simulink model "parallel_phase_voltages_per_switching_state_6"  (R2022a)
settings: Solver=FixedStepDiscrete  StartTime=0.0  StopTime=10.0  RelTol=1e-3
values from neighbouring files (symbols this model uses):
  f_c = 100000    [MPC_params.m]
  Rt = 1e-8    (= 1e-08)    [MPC_params.m]
  u_dc = 565    [MPC_params.m]
libraries: simulink x2, hdlsllib x2
(part 2 of 4)

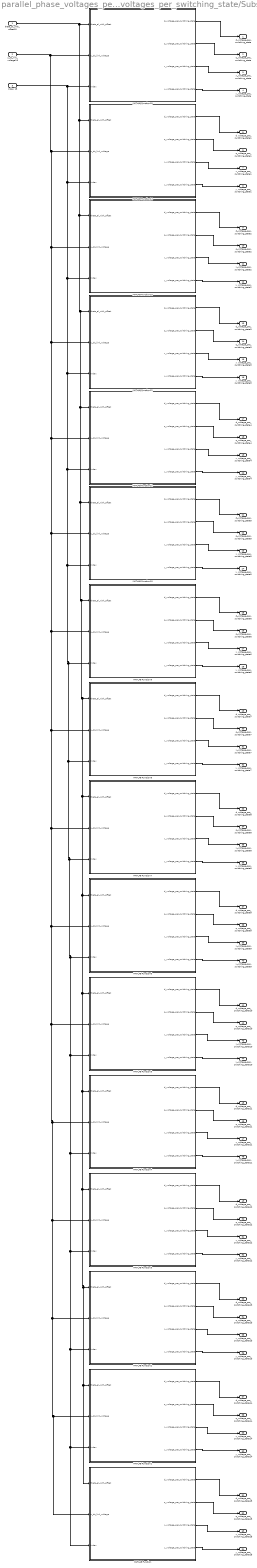
== system parallel_phase_voltages_per_switching_state_6/Phase_voltages_per_switching_state/Subsystem ==
  theta_el_with_offset15 : Inport
  u_dc_link_voltage15 : Inport  Port=2
  Index 15 : Inport  Port=3
  MATLAB Function : MATLAB Function  TreatAsAtomicUnit=on
  MATLAB Function1 : MATLAB Function  TreatAsAtomicUnit=on
  MATLAB Function10 : MATLAB Function  TreatAsAtomicUnit=on
  MATLAB Function11 : MATLAB Function  TreatAsAtomicUnit=on
  MATLAB Function12 : MATLAB Function  TreatAsAtomicUnit=on
  MATLAB Function13 : MATLAB Function  TreatAsAtomicUnit=on
  MATLAB Function14 : MATLAB Function  TreatAsAtomicUnit=on
  MATLAB Function15 : MATLAB Function  TreatAsAtomicUnit=on
  MATLAB Function2 : MATLAB Function  TreatAsAtomicUnit=on
  MATLAB Function3 : MATLAB Function  TreatAsAtomicUnit=on
  MATLAB Function4 : MATLAB Function  TreatAsAtomicUnit=on
  MATLAB Function5 : MATLAB Function  TreatAsAtomicUnit=on
  MATLAB Function6 : MATLAB Function  TreatAsAtomicUnit=on
  MATLAB Function7 : MATLAB Function  TreatAsAtomicUnit=on
  MATLAB Function8 : MATLAB Function  TreatAsAtomicUnit=on
  MATLAB Function9 : MATLAB Function  TreatAsAtomicUnit=on
  d_voltage_per_switching_state : Outport
  q_voltage_per_switching_state : Outport  Port=2
  x_voltage_per_switching_state : Outport  Port=3
  y_voltage_per_switching_state : Outport  Port=4
  d_voltage_per_switching_state1 : Outport  Port=5
  q_voltage_per_switching_state1 : Outport  Port=6
  x_voltage_per_switching_state1 : Outport  Port=7
  y_voltage_per_switching_state1 : Outport  Port=8
  d_voltage_per_switching_state2 : Outport  Port=9
  q_voltage_per_switching_state2 : Outport  Port=10
  x_voltage_per_switching_state2 : Outport  Port=11
  y_voltage_per_switching_state2 : Outport  Port=12
  d_voltage_per_switching_state3 : Outport  Port=13
  q_voltage_per_switching_state3 : Outport  Port=14
  x_voltage_per_switching_state3 : Outport  Port=15
  y_voltage_per_switching_state3 : Outport  Port=16
  d_voltage_per_switching_state4 : Outport  Port=17
  q_voltage_per_switching_state4 : Outport  Port=18
  x_voltage_per_switching_state4 : Outport  Port=19
  y_voltage_per_switching_state4 : Outport  Port=20
  d_voltage_per_switching_state5 : Outport  Port=21
  q_voltage_per_switching_state5 : Outport  Port=22
  x_voltage_per_switching_state5 : Outport  Port=23
  y_voltage_per_switching_state5 : Outport  Port=24
  d_voltage_per_switching_state6 : Outport  Port=25
  q_voltage_per_switching_state6 : Outport  Port=26
  x_voltage_per_switching_state6 : Outport  Port=27
  y_voltage_per_switching_state6 : Outport  Port=28
  d_voltage_per_switching_state7 : Outport  Port=29
  q_voltage_per_switching_state7 : Outport  Port=30
  x_voltage_per_switching_state7 : Outport  Port=31
  y_voltage_per_switching_state7 : Outport  Port=32
  d_voltage_per_switching_state8 : Outport  Port=33
  q_voltage_per_switching_state8 : Outport  Port=34
  x_voltage_per_switching_state8 : Outport  Port=35
  y_voltage_per_switching_state8 : Outport  Port=36
  d_voltage_per_switching_state9 : Outport  Port=37
  q_voltage_per_switching_state9 : Outport  Port=38
  x_voltage_per_switching_state9 : Outport  Port=39
  y_voltage_per_switching_state9 : Outport  Port=40
  d_voltage_per_switching_state10 : Outport  Port=41
  q_voltage_per_switching_state10 : Outport  Port=42
  x_voltage_per_switching_state10 : Outport  Port=43
  y_voltage_per_switching_state10 : Outport  Port=44
  d_voltage_per_switching_state11 : Outport  Port=45
  q_voltage_per_switching_state11 : Outport  Port=46
  x_voltage_per_switching_state11 : Outport  Port=47
  y_voltage_per_switching_state11 : Outport  Port=48
  d_voltage_per_switching_state12 : Outport  Port=49
  q_voltage_per_switching_state12 : Outport  Port=50
  x_voltage_per_switching_state12 : Outport  Port=51
  y_voltage_per_switching_state12 : Outport  Port=52
  d_voltage_per_switching_state13 : Outport  Port=53
  q_voltage_per_switching_state13 : Outport  Port=54
  x_voltage_per_switching_state13 : Outport  Port=55
  y_voltage_per_switching_state13 : Outport  Port=56
  d_voltage_per_switching_state14 : Outport  Port=57
  q_voltage_per_switching_state14 : Outport  Port=58
  x_voltage_per_switching_state14 : Outport  Port=59
  y_voltage_per_switching_state14 : Outport  Port=60
  d_voltage_per_switching_state15 : Outport  Port=61
  q_voltage_per_switching_state15 : Outport  Port=62
  x_voltage_per_switching_state15 : Outport  Port=63
  y_voltage_per_switching_state15 : Outport  Port=64
  wires:
  MATLAB Function4/1(d_voltage_per_switching_state) -> d_voltage_per_switching_state11/1
  MATLAB Function11/4(y_voltage_per_switching_state) -> y_voltage_per_switching_state4/1
  MATLAB Function3/2(q_voltage_per_switching_state) -> q_voltage_per_switching_state12/1
  MATLAB Function3/4(y_voltage_per_switching_state) -> y_voltage_per_switching_state12/1
  MATLAB Function10/3(x_voltage_per_switching_state) -> x_voltage_per_switching_state5/1
  MATLAB Function8/1(d_voltage_per_switching_state) -> d_voltage_per_switching_state7/1
  MATLAB Function8/2(q_voltage_per_switching_state) -> q_voltage_per_switching_state7/1
  MATLAB Function3/1(d_voltage_per_switching_state) -> d_voltage_per_switching_state12/1
  MATLAB Function11/1(d_voltage_per_switching_state) -> d_voltage_per_switching_state4/1
  theta_el_with_offset15/1 -> MATLAB Function/1(theta_el_with_offset), MATLAB Function1/1(theta_el_with_offset), MATLAB Function2/1(theta_el_with_offset), MATLAB Function3/1(theta_el_with_offset), MATLAB Function4/1(theta_el_with_offset), MATLAB Function5/1(theta_el_with_offset), MATLAB Function6/1(theta_el_with_offset), MATLAB Function7/1(theta_el_with_offset), MATLAB Function8/1(theta_el_with_offset), MATLAB Function9/1(theta_el_with_offset), MATLAB Function10/1(theta_el_with_offset), MATLAB Function11/1(theta_el_with_offset), MATLAB Function12/1(theta_el_with_offset), MATLAB Function13/1(theta_el_with_offset), MATLAB Function14/1(theta_el_with_offset), MATLAB Function15/1(theta_el_with_offset)
  MATLAB Function12/3(x_voltage_per_switching_state) -> x_voltage_per_switching_state3/1
  MATLAB Function15/2(q_voltage_per_switching_state) -> q_voltage_per_switching_state/1
  MATLAB Function8/3(x_voltage_per_switching_state) -> x_voltage_per_switching_state7/1
  MATLAB Function/1(d_voltage_per_switching_state) -> d_voltage_per_switching_state15/1
  MATLAB Function11/3(x_voltage_per_switching_state) -> x_voltage_per_switching_state4/1
  MATLAB Function10/4(y_voltage_per_switching_state) -> y_voltage_per_switching_state5/1
  MATLAB Function4/3(x_voltage_per_switching_state) -> x_voltage_per_switching_state11/1
  MATLAB Function11/2(q_voltage_per_switching_state) -> q_voltage_per_switching_state4/1
  MATLAB Function12/1(d_voltage_per_switching_state) -> d_voltage_per_switching_state3/1
  MATLAB Function2/1(d_voltage_per_switching_state) -> d_voltage_per_switching_state13/1
  MATLAB Function12/4(y_voltage_per_switching_state) -> y_voltage_per_switching_state3/1
  MATLAB Function/3(x_voltage_per_switching_state) -> x_voltage_per_switching_state15/1
  MATLAB Function13/2(q_voltage_per_switching_state) -> q_voltage_per_switching_state2/1
  MATLAB Function10/1(d_voltage_per_switching_state) -> d_voltage_per_switching_state5/1
  MATLAB Function10/2(q_voltage_per_switching_state) -> q_voltage_per_switching_state5/1
  MATLAB Function4/4(y_voltage_per_switching_state) -> y_voltage_per_switching_state11/1
  MATLAB Function3/3(x_voltage_per_switching_state) -> x_voltage_per_switching_state12/1
  MATLAB Function13/4(y_voltage_per_switching_state) -> y_voltage_per_switching_state2/1
  MATLAB Function8/4(y_voltage_per_switching_state) -> y_voltage_per_switching_state7/1
  MATLAB Function13/1(d_voltage_per_switching_state) -> d_voltage_per_switching_state2/1
  MATLAB Function13/3(x_voltage_per_switching_state) -> x_voltage_per_switching_state2/1
  MATLAB Function1/4(y_voltage_per_switching_state) -> y_voltage_per_switching_state14/1
  MATLAB Function1/1(d_voltage_per_switching_state) -> d_voltage_per_switching_state14/1
  MATLAB Function12/2(q_voltage_per_switching_state) -> q_voltage_per_switching_state3/1
  MATLAB Function4/2(q_voltage_per_switching_state) -> q_voltage_per_switching_state11/1
  MATLAB Function6/2(q_voltage_per_switching_state) -> q_voltage_per_switching_state9/1
  MATLAB Function5/3(x_voltage_per_switching_state) -> x_voltage_per_switching_state10/1
  MATLAB Function6/3(x_voltage_per_switching_state) -> x_voltage_per_switching_state9/1
  MATLAB Function6/1(d_voltage_per_switching_state) -> d_voltage_per_switching_state9/1
  MATLAB Function6/4(y_voltage_per_switching_state) -> y_voltage_per_switching_state9/1
  MATLAB Function15/1(d_voltage_per_switching_state) -> d_voltage_per_switching_state/1
  MATLAB Function15/4(y_voltage_per_switching_state) -> y_voltage_per_switching_state/1
  MATLAB Function15/3(x_voltage_per_switching_state) -> x_voltage_per_switching_state/1
  MATLAB Function/4(y_voltage_per_switching_state) -> y_voltage_per_switching_state15/1
  MATLAB Function/2(q_voltage_per_switching_state) -> q_voltage_per_switching_state15/1
  u_dc_link_voltage15/1 -> MATLAB Function/2(u_dc_link_voltage), MATLAB Function1/2(u_dc_link_voltage), MATLAB Function2/2(u_dc_link_voltage), MATLAB Function3/2(u_dc_link_voltage), MATLAB Function4/2(u_dc_link_voltage), MATLAB Function5/2(u_dc_link_voltage), MATLAB Function6/2(u_dc_link_voltage), MATLAB Function7/2(u_dc_link_voltage), MATLAB Function8/2(u_dc_link_voltage), MATLAB Function9/2(u_dc_link_voltage), MATLAB Function10/2(u_dc_link_voltage), MATLAB Function11/2(u_dc_link_voltage), MATLAB Function12/2(u_dc_link_voltage), MATLAB Function13/2(u_dc_link_voltage), MATLAB Function14/2(u_dc_link_voltage), MATLAB Function15/2(u_dc_link_voltage)
  MATLAB Function14/4(y_voltage_per_switching_state) -> y_voltage_per_switching_state1/1
  MATLAB Function2/2(q_voltage_per_switching_state) -> q_voltage_per_switching_state13/1
  MATLAB Function14/3(x_voltage_per_switching_state) -> x_voltage_per_switching_state1/1
  MATLAB Function14/1(d_voltage_per_switching_state) -> d_voltage_per_switching_state1/1
  MATLAB Function14/2(q_voltage_per_switching_state) -> q_voltage_per_switching_state1/1
  Index 15/1 -> MATLAB Function15/3(Index), MATLAB Function10/3(Index), MATLAB Function8/3(Index), MATLAB Function/3(Index), MATLAB Function1/3(Index), MATLAB Function2/3(Index), MATLAB Function3/3(Index), MATLAB Function4/3(Index), MATLAB Function5/3(Index), MATLAB Function6/3(Index), MATLAB Function7/3(Index), MATLAB Function9/3(Index), MATLAB Function11/3(Index), MATLAB Function12/3(Index), MATLAB Function13/3(Index), MATLAB Function14/3(Index)
  MATLAB Function1/2(q_voltage_per_switching_state) -> q_voltage_per_switching_state14/1
  MATLAB Function1/3(x_voltage_per_switching_state) -> x_voltage_per_switching_state14/1
  MATLAB Function9/3(x_voltage_per_switching_state) -> x_voltage_per_switching_state6/1
  MATLAB Function9/2(q_voltage_per_switching_state) -> q_voltage_per_switching_state6/1
  MATLAB Function9/1(d_voltage_per_switching_state) -> d_voltage_per_switching_state6/1
  MATLAB Function9/4(y_voltage_per_switching_state) -> y_voltage_per_switching_state6/1
  MATLAB Function7/1(d_voltage_per_switching_state) -> d_voltage_per_switching_state8/1
  MATLAB Function7/4(y_voltage_per_switching_state) -> y_voltage_per_switching_state8/1
  MATLAB Function7/2(q_voltage_per_switching_state) -> q_voltage_per_switching_state8/1
  MATLAB Function7/3(x_voltage_per_switching_state) -> x_voltage_per_switching_state8/1
  MATLAB Function5/2(q_voltage_per_switching_state) -> q_voltage_per_switching_state10/1
  MATLAB Function5/1(d_voltage_per_switching_state) -> d_voltage_per_switching_state10/1
  MATLAB Function5/4(y_voltage_per_switching_state) -> y_voltage_per_switching_state10/1
  MATLAB Function2/3(x_voltage_per_switching_state) -> x_voltage_per_switching_state13/1
  MATLAB Function2/4(y_voltage_per_switching_state) -> y_voltage_per_switching_state13/1

== matlab function parallel_phase_voltages_per_switching_state_6/Phase_voltages_per_switching_state/Subsystem/MATLAB Function8 ==
  data: theta_el_with_offset input; d_voltage_per_switching_state output; u_dc_link_voltage input; Index input; q_voltage_per_switching_state output; x_voltage_per_switching_state output; y_voltage_per_switching_state output
function [d_voltage_per_switching_state, q_voltage_per_switching_state, x_voltage_per_switching_state, y_voltage_per_switching_state] = fcn(theta_el_with_offset, u_dc_link_voltage, Index)
      
        % Initial condition
            Index = Index+1+28;

    
        % Swichtingstates factors alpha beta x y
        Factors_alpha_beta_x_y = single([0	    0.333333333333333	-0.166666666666667	 0.166666666666667	-0.166666666666667	 0.166666666666667	-0.333333333333333	0	 0.288675134594813	0.622008467928146	 0.122008467928146  	0.455341801261480	 0.122008467928146	 0.455341801261480	-0.0446581987385205  0.288675134594813	-0.288675134594813	0.0446581987385205	-0.455341801261480	-0.122008467928146	-0.455341801261480	-0.122008467928146	-0.622008467928146	-0.288675134594813	0	                0.333333333333333	-0.166666666666667  	0.166666666666667	-0.166666666666667	 0.166666666666667	 -0.333333333333333	0	                 0	                 0.333333333333333	-0.166666666666667	  0.166666666666667	    -0.166666666666667	  0.166666666666667	    -0.333333333333333	 0	                 0.288675134594813	 0.622008467928146	 0.122008467928146	 0.455341801261480	 0.122008467928146	 0.455341801261480	-0.0446581987385205  0.288675134594813	-0.288675134594813	 0.0446581987385205  -0.455341801261480	  -0.122008467928146	-0.455341801261480	-0.122008467928146	-0.622008467928146	-0.288675134594813	0	0.333333333333333	-0.166666666666667	 0.166666666666667	-0.166666666666667	 0.166666666666667	-0.333333333333333	0;
                                         0	    0                    0.288675134594813	 0.288675134594813	-0.288675134594813	-0.288675134594813	 0	                0	 0.166666666666667	0.166666666666667	 0.455341801261480  	0.455341801261480	-0.122008467928146	-0.122008467928146	 0.166666666666667	 0.166666666666667	 0.166666666666667	0.166666666666667	 0.455341801261480   0.455341801261480	-0.122008467928146	-0.122008467928146	 0.166666666666667	 0.166666666666667	0.333333333333333	0.333333333333333	 0.622008467928146	    0.622008467928146	 0.0446581987385205	 0.0446581987385205	  0.333333333333333	0.333333333333333	-0.333333333333333	-0.333333333333333	-0.0446581987385205	 -0.0446581987385205	-0.622008467928146	 -0.622008467928146	    -0.333333333333333	-0.333333333333333	-0.166666666666667	-0.166666666666667	 0.122008467928146	 0.122008467928146	-0.455341801261480	-0.455341801261480	-0.166666666666667	-0.166666666666667	-0.166666666666667	-0.166666666666667	  0.122008467928146	   0.122008467928146	-0.455341801261480	-0.455341801261480	-0.166666666666667	-0.166666666666667	0	0	                 0.288675134594813	 0.288675134594813	-0.288675134594813	-0.288675134594813	 0	                0;
                                         0	    0.333333333333333	-0.166666666666667	 0.166666666666667	-0.166666666666667	 0.166666666666667	-0.333333333333333	0	-0.288675134594813	0.0446581987385205	-0.455341801261480	   -0.122008467928146	-0.455341801261480	-0.122008467928146	-0.622008467928146	-0.288675134594813	 0.288675134594813	0.622008467928146	 0.122008467928146	 0.455341801261480   0.122008467928146	 0.455341801261480	-0.0446581987385205	 0.288675134594813	0	                0.333333333333333	-0.166666666666667	    0.166666666666667	-0.166666666666667	 0.166666666666667	 -0.333333333333333	0	                 0	                 0.333333333333333	-0.166666666666667	  0.166666666666667	    -0.166666666666667	  0.166666666666667	    -0.333333333333333	 0	                -0.288675134594813	 0.0446581987385205	-0.455341801261480	-0.122008467928146	-0.455341801261480	-0.122008467928146	-0.622008467928146	-0.288675134594813	 0.288675134594813	 0.622008467928146	  0.122008467928146	   0.455341801261480	 0.122008467928146	 0.455341801261480	-0.0446581987385205  0.288675134594813	0	0.333333333333333	-0.166666666666667	 0.166666666666667	-0.166666666666667	 0.166666666666667	-0.333333333333333	0;
                                         0	    0	                -0.288675134594813	-0.288675134594813	 0.288675134594813	 0.288675134594813	 0              	0	 0.166666666666667	0.166666666666667	-0.122008467928146     -0.122008467928146	 0.455341801261480	 0.455341801261480	 0.166666666666667	 0.166666666666667	 0.166666666666667	0.166666666666667	-0.122008467928146	-0.122008467928146	 0.455341801261480	 0.455341801261480	 0.166666666666667	 0.166666666666667	0.333333333333333	0.333333333333333	 0.0446581987385205 	0.0446581987385205	 0.622008467928146	 0.622008467928146	  0.333333333333333	0.333333333333333	-0.333333333333333	-0.333333333333333	-0.622008467928146	 -0.622008467928146	    -0.0446581987385205	 -0.0446581987385205	-0.333333333333333	-0.333333333333333	-0.166666666666667	-0.166666666666667	-0.455341801261480	-0.455341801261480	 0.122008467928146	 0.122008467928146	-0.166666666666667	-0.166666666666667	-0.166666666666667	-0.166666666666667	 -0.455341801261480	  -0.455341801261480	 0.122008467928146	 0.122008467928146	-0.166666666666667	-0.166666666666667	0	0	                -0.288675134594813	-0.288675134594813	 0.288675134594813	 0.288675134594813	 0	                0]);
        
        % Park-Transformation of the switchingstates factors
        Factors_d_q_x_y =single(zeros(4,1));
    
        Factors_d_q_x_y(3,1) = Factors_alpha_beta_x_y(3,Index);
        Factors_d_q_x_y(4,1) = Factors_alpha_beta_x_y(4,Index);
    
        cos_theta_el = single(cos(theta_el_with_offset));
        sin_theta_el = single(sin(theta_el_with_offset));
       
        Factors_d_q_x_y(1,1) = cos_theta_el*Factors_alpha_beta_x_y(1,Index)+sin_theta_el*Factors_alpha_beta_x_y(2,Index);
        Factors_d_q_x_y(2,1) = -sin_theta_el*Factors_alpha_beta_x_y(1,Index)+cos_theta_el*Factors_alpha_beta_x_y(2,Index);
    
        %Calculation of the voltages per switching state in alpha beta coordinates
        d_q_x_y_voltages_per_switching_state = single(u_dc_link_voltage*Factors_d_q_x_y);
    
        d_voltage_per_switching_state = d_q_x_y_voltages_per_switching_state(1,1);
        q_voltage_per_switching_state = d_q_x_y_voltages_per_switching_state(2,1);
        x_voltage_per_switching_state = d_q_x_y_voltages_per_switching_state(3,1);
        y_voltage_per_switching_state = d_q_x_y_voltages_per_switching_state(4,1);
    

end

== matlab function parallel_phase_voltages_per_switching_state_6/Phase_voltages_per_switching_state/Subsystem/MATLAB Function9 ==
  data: theta_el_with_offset input; d_voltage_per_switching_state output; u_dc_link_voltage input; Index input; q_voltage_per_switching_state output; x_voltage_per_switching_state output; y_voltage_per_switching_state output
function [d_voltage_per_switching_state, q_voltage_per_switching_state, x_voltage_per_switching_state, y_voltage_per_switching_state] = fcn(theta_el_with_offset, u_dc_link_voltage, Index)
      
        % Initial condition
            Index = Index+1+24;

    
        % Swichtingstates factors alpha beta x y
        Factors_alpha_beta_x_y = single([0	    0.333333333333333	-0.166666666666667	 0.166666666666667	-0.166666666666667	 0.166666666666667	-0.333333333333333	0	 0.288675134594813	0.622008467928146	 0.122008467928146  	0.455341801261480	 0.122008467928146	 0.455341801261480	-0.0446581987385205  0.288675134594813	-0.288675134594813	0.0446581987385205	-0.455341801261480	-0.122008467928146	-0.455341801261480	-0.122008467928146	-0.622008467928146	-0.288675134594813	0	                0.333333333333333	-0.166666666666667  	0.166666666666667	-0.166666666666667	 0.166666666666667	 -0.333333333333333	0	                 0	                 0.333333333333333	-0.166666666666667	  0.166666666666667	    -0.166666666666667	  0.166666666666667	    -0.333333333333333	 0	                 0.288675134594813	 0.622008467928146	 0.122008467928146	 0.455341801261480	 0.122008467928146	 0.455341801261480	-0.0446581987385205  0.288675134594813	-0.288675134594813	 0.0446581987385205  -0.455341801261480	  -0.122008467928146	-0.455341801261480	-0.122008467928146	-0.622008467928146	-0.288675134594813	0	0.333333333333333	-0.166666666666667	 0.166666666666667	-0.166666666666667	 0.166666666666667	-0.333333333333333	0;
                                         0	    0                    0.288675134594813	 0.288675134594813	-0.288675134594813	-0.288675134594813	 0	                0	 0.166666666666667	0.166666666666667	 0.455341801261480  	0.455341801261480	-0.122008467928146	-0.122008467928146	 0.166666666666667	 0.166666666666667	 0.166666666666667	0.166666666666667	 0.455341801261480   0.455341801261480	-0.122008467928146	-0.122008467928146	 0.166666666666667	 0.166666666666667	0.333333333333333	0.333333333333333	 0.622008467928146	    0.622008467928146	 0.0446581987385205	 0.0446581987385205	  0.333333333333333	0.333333333333333	-0.333333333333333	-0.333333333333333	-0.0446581987385205	 -0.0446581987385205	-0.622008467928146	 -0.622008467928146	    -0.333333333333333	-0.333333333333333	-0.166666666666667	-0.166666666666667	 0.122008467928146	 0.122008467928146	-0.455341801261480	-0.455341801261480	-0.166666666666667	-0.166666666666667	-0.166666666666667	-0.166666666666667	  0.122008467928146	   0.122008467928146	-0.455341801261480	-0.455341801261480	-0.166666666666667	-0.166666666666667	0	0	                 0.288675134594813	 0.288675134594813	-0.288675134594813	-0.288675134594813	 0	                0;
                                         0	    0.333333333333333	-0.166666666666667	 0.166666666666667	-0.166666666666667	 0.166666666666667	-0.333333333333333	0	-0.288675134594813	0.0446581987385205	-0.455341801261480	   -0.122008467928146	-0.455341801261480	-0.122008467928146	-0.622008467928146	-0.288675134594813	 0.288675134594813	0.622008467928146	 0.122008467928146	 0.455341801261480   0.122008467928146	 0.455341801261480	-0.0446581987385205	 0.288675134594813	0	                0.333333333333333	-0.166666666666667	    0.166666666666667	-0.166666666666667	 0.166666666666667	 -0.333333333333333	0	                 0	                 0.333333333333333	-0.166666666666667	  0.166666666666667	    -0.166666666666667	  0.166666666666667	    -0.333333333333333	 0	                -0.288675134594813	 0.0446581987385205	-0.455341801261480	-0.122008467928146	-0.455341801261480	-0.122008467928146	-0.622008467928146	-0.288675134594813	 0.288675134594813	 0.622008467928146	  0.122008467928146	   0.455341801261480	 0.122008467928146	 0.455341801261480	-0.0446581987385205  0.288675134594813	0	0.333333333333333	-0.166666666666667	 0.166666666666667	-0.166666666666667	 0.166666666666667	-0.333333333333333	0;
                                         0	    0	                -0.288675134594813	-0.288675134594813	 0.288675134594813	 0.288675134594813	 0              	0	 0.166666666666667	0.166666666666667	-0.122008467928146     -0.122008467928146	 0.455341801261480	 0.455341801261480	 0.166666666666667	 0.166666666666667	 0.166666666666667	0.166666666666667	-0.122008467928146	-0.122008467928146	 0.455341801261480	 0.455341801261480	 0.166666666666667	 0.166666666666667	0.333333333333333	0.333333333333333	 0.0446581987385205 	0.0446581987385205	 0.622008467928146	 0.622008467928146	  0.333333333333333	0.333333333333333	-0.333333333333333	-0.333333333333333	-0.622008467928146	 -0.622008467928146	    -0.0446581987385205	 -0.0446581987385205	-0.333333333333333	-0.333333333333333	-0.166666666666667	-0.166666666666667	-0.455341801261480	-0.455341801261480	 0.122008467928146	 0.122008467928146	-0.166666666666667	-0.166666666666667	-0.166666666666667	-0.166666666666667	 -0.455341801261480	  -0.455341801261480	 0.122008467928146	 0.122008467928146	-0.166666666666667	-0.166666666666667	0	0	                -0.288675134594813	-0.288675134594813	 0.288675134594813	 0.288675134594813	 0	                0]);
        
        % Park-Transformation of the switchingstates factors
        Factors_d_q_x_y =single(zeros(4,1));
    
        Factors_d_q_x_y(3,1) = Factors_alpha_beta_x_y(3,Index);
        Factors_d_q_x_y(4,1) = Factors_alpha_beta_x_y(4,Index);
    
        cos_theta_el = single(cos(theta_el_with_offset));
        sin_theta_el = single(sin(theta_el_with_offset));
       
        Factors_d_q_x_y(1,1) = cos_theta_el*Factors_alpha_beta_x_y(1,Index)+sin_theta_el*Factors_alpha_beta_x_y(2,Index);
        Factors_d_q_x_y(2,1) = -sin_theta_el*Factors_alpha_beta_x_y(1,Index)+cos_theta_el*Factors_alpha_beta_x_y(2,Index);
    
        %Calculation of the voltages per switching state in alpha beta coordinates
        d_q_x_y_voltages_per_switching_state = single(u_dc_link_voltage*Factors_d_q_x_y);
    
        d_voltage_per_switching_state = d_q_x_y_voltages_per_switching_state(1,1);
        q_voltage_per_switching_state = d_q_x_y_voltages_per_switching_state(2,1);
        x_voltage_per_switching_state = d_q_x_y_voltages_per_switching_state(3,1);
        y_voltage_per_switching_state = d_q_x_y_voltages_per_switching_state(4,1);
    

end

== matlab function parallel_phase_voltages_per_switching_state_6/Phase_voltages_per_switching_state/Subsystem/MATLAB Function10 ==
  data: theta_el_with_offset input; d_voltage_per_switching_state output; u_dc_link_voltage input; Index input; q_voltage_per_switching_state output; x_voltage_per_switching_state output; y_voltage_per_switching_state output
function [d_voltage_per_switching_state, q_voltage_per_switching_state, x_voltage_per_switching_state, y_voltage_per_switching_state] = fcn(theta_el_with_offset, u_dc_link_voltage, Index)
      
        % Initial condition
            Index = Index+1+20;

        % Swichtingstates factors alpha beta x y
        Factors_alpha_beta_x_y = single([0	    0.333333333333333	-0.166666666666667	 0.166666666666667	-0.166666666666667	 0.166666666666667	-0.333333333333333	0	 0.288675134594813	0.622008467928146	 0.122008467928146  	0.455341801261480	 0.122008467928146	 0.455341801261480	-0.0446581987385205  0.288675134594813	-0.288675134594813	0.0446581987385205	-0.455341801261480	-0.122008467928146	-0.455341801261480	-0.122008467928146	-0.622008467928146	-0.288675134594813	0	                0.333333333333333	-0.166666666666667  	0.166666666666667	-0.166666666666667	 0.166666666666667	 -0.333333333333333	0	                 0	                 0.333333333333333	-0.166666666666667	  0.166666666666667	    -0.166666666666667	  0.166666666666667	    -0.333333333333333	 0	                 0.288675134594813	 0.622008467928146	 0.122008467928146	 0.455341801261480	 0.122008467928146	 0.455341801261480	-0.0446581987385205  0.288675134594813	-0.288675134594813	 0.0446581987385205  -0.455341801261480	  -0.122008467928146	-0.455341801261480	-0.122008467928146	-0.622008467928146	-0.288675134594813	0	0.333333333333333	-0.166666666666667	 0.166666666666667	-0.166666666666667	 0.166666666666667	-0.333333333333333	0;
                                         0	    0                    0.288675134594813	 0.288675134594813	-0.288675134594813	-0.288675134594813	 0	                0	 0.166666666666667	0.166666666666667	 0.455341801261480  	0.455341801261480	-0.122008467928146	-0.122008467928146	 0.166666666666667	 0.166666666666667	 0.166666666666667	0.166666666666667	 0.455341801261480   0.455341801261480	-0.122008467928146	-0.122008467928146	 0.166666666666667	 0.166666666666667	0.333333333333333	0.333333333333333	 0.622008467928146	    0.622008467928146	 0.0446581987385205	 0.0446581987385205	  0.333333333333333	0.333333333333333	-0.333333333333333	-0.333333333333333	-0.0446581987385205	 -0.0446581987385205	-0.622008467928146	 -0.622008467928146	    -0.333333333333333	-0.333333333333333	-0.166666666666667	-0.166666666666667	 0.122008467928146	 0.122008467928146	-0.455341801261480	-0.455341801261480	-0.166666666666667	-0.166666666666667	-0.166666666666667	-0.166666666666667	  0.122008467928146	   0.122008467928146	-0.455341801261480	-0.455341801261480	-0.166666666666667	-0.166666666666667	0	0	                 0.288675134594813	 0.288675134594813	-0.288675134594813	-0.288675134594813	 0	                0;
                                         0	    0.333333333333333	-0.166666666666667	 0.166666666666667	-0.166666666666667	 0.166666666666667	-0.333333333333333	0	-0.288675134594813	0.0446581987385205	-0.455341801261480	   -0.122008467928146	-0.455341801261480	-0.122008467928146	-0.622008467928146	-0.288675134594813	 0.288675134594813	0.622008467928146	 0.122008467928146	 0.455341801261480   0.122008467928146	 0.455341801261480	-0.0446581987385205	 0.288675134594813	0	                0.333333333333333	-0.166666666666667	    0.166666666666667	-0.166666666666667	 0.166666666666667	 -0.333333333333333	0	                 0	                 0.333333333333333	-0.166666666666667	  0.166666666666667	    -0.166666666666667	  0.166666666666667	    -0.333333333333333	 0	                -0.288675134594813	 0.0446581987385205	-0.455341801261480	-0.122008467928146	-0.455341801261480	-0.122008467928146	-0.622008467928146	-0.288675134594813	 0.288675134594813	 0.622008467928146	  0.122008467928146	   0.455341801261480	 0.122008467928146	 0.455341801261480	-0.0446581987385205  0.288675134594813	0	0.333333333333333	-0.166666666666667	 0.166666666666667	-0.166666666666667	 0.166666666666667	-0.333333333333333	0;
                                         0	    0	                -0.288675134594813	-0.288675134594813	 0.288675134594813	 0.288675134594813	 0              	0	 0.166666666666667	0.166666666666667	-0.122008467928146     -0.122008467928146	 0.455341801261480	 0.455341801261480	 0.166666666666667	 0.166666666666667	 0.166666666666667	0.166666666666667	-0.122008467928146	-0.122008467928146	 0.455341801261480	 0.455341801261480	 0.166666666666667	 0.166666666666667	0.333333333333333	0.333333333333333	 0.0446581987385205 	0.0446581987385205	 0.622008467928146	 0.622008467928146	  0.333333333333333	0.333333333333333	-0.333333333333333	-0.333333333333333	-0.622008467928146	 -0.622008467928146	    -0.0446581987385205	 -0.0446581987385205	-0.333333333333333	-0.333333333333333	-0.166666666666667	-0.166666666666667	-0.455341801261480	-0.455341801261480	 0.122008467928146	 0.122008467928146	-0.166666666666667	-0.166666666666667	-0.166666666666667	-0.166666666666667	 -0.455341801261480	  -0.455341801261480	 0.122008467928146	 0.122008467928146	-0.166666666666667	-0.166666666666667	0	0	                -0.288675134594813	-0.288675134594813	 0.288675134594813	 0.288675134594813	 0	                0]);
        
        % Park-Transformation of the switchingstates factors
        Factors_d_q_x_y =single(zeros(4,1));
    
        Factors_d_q_x_y(3,1) = Factors_alpha_beta_x_y(3,Index);
        Factors_d_q_x_y(4,1) = Factors_alpha_beta_x_y(4,Index);
    
        cos_theta_el = single(cos(theta_el_with_offset));
        sin_theta_el = single(sin(theta_el_with_offset));
       
        Factors_d_q_x_y(1,1) = cos_theta_el*Factors_alpha_beta_x_y(1,Index)+sin_theta_el*Factors_alpha_beta_x_y(2,Index);
        Factors_d_q_x_y(2,1) = -sin_theta_el*Factors_alpha_beta_x_y(1,Index)+cos_theta_el*Factors_alpha_beta_x_y(2,Index);
    
        %Calculation of the voltages per switching state in alpha beta coordinates
        d_q_x_y_voltages_per_switching_state = single(u_dc_link_voltage*Factors_d_q_x_y);
    
        d_voltage_per_switching_state = d_q_x_y_voltages_per_switching_state(1,1);
        q_voltage_per_switching_state = d_q_x_y_voltages_per_switching_state(2,1);
        x_voltage_per_switching_state = d_q_x_y_voltages_per_switching_state(3,1);
        y_voltage_per_switching_state = d_q_x_y_voltages_per_switching_state(4,1);
    

end

== matlab function parallel_phase_voltages_per_switching_state_6/Phase_voltages_per_switching_state/Subsystem/MATLAB Function ==
  data: theta_el_with_offset input; d_voltage_per_switching_state output; u_dc_link_voltage input; Index input; q_voltage_per_switching_state output; x_voltage_per_switching_state output; y_voltage_per_switching_state output
function [d_voltage_per_switching_state, q_voltage_per_switching_state, x_voltage_per_switching_state, y_voltage_per_switching_state] = fcn(theta_el_with_offset, u_dc_link_voltage, Index)
      
        % Initial condition
            Index = Index+1+60;

    
        % Swichtingstates factors alpha beta x y
        Factors_alpha_beta_x_y = single([0	    0.333333333333333	-0.166666666666667	 0.166666666666667	-0.166666666666667	 0.166666666666667	-0.333333333333333	0	 0.288675134594813	0.622008467928146	 0.122008467928146  	0.455341801261480	 0.122008467928146	 0.455341801261480	-0.0446581987385205  0.288675134594813	-0.288675134594813	0.0446581987385205	-0.455341801261480	-0.122008467928146	-0.455341801261480	-0.122008467928146	-0.622008467928146	-0.288675134594813	0	                0.333333333333333	-0.166666666666667  	0.166666666666667	-0.166666666666667	 0.166666666666667	 -0.333333333333333	0	                 0	                 0.333333333333333	-0.166666666666667	  0.166666666666667	    -0.166666666666667	  0.166666666666667	    -0.333333333333333	 0	                 0.288675134594813	 0.622008467928146	 0.122008467928146	 0.455341801261480	 0.122008467928146	 0.455341801261480	-0.0446581987385205  0.288675134594813	-0.288675134594813	 0.0446581987385205  -0.455341801261480	  -0.122008467928146	-0.455341801261480	-0.122008467928146	-0.622008467928146	-0.288675134594813	0	0.333333333333333	-0.166666666666667	 0.166666666666667	-0.166666666666667	 0.166666666666667	-0.333333333333333	0;
                                         0	    0                    0.288675134594813	 0.288675134594813	-0.288675134594813	-0.288675134594813	 0	                0	 0.166666666666667	0.166666666666667	 0.455341801261480  	0.455341801261480	-0.122008467928146	-0.122008467928146	 0.166666666666667	 0.166666666666667	 0.166666666666667	0.166666666666667	 0.455341801261480   0.455341801261480	-0.122008467928146	-0.122008467928146	 0.166666666666667	 0.166666666666667	0.333333333333333	0.333333333333333	 0.622008467928146	    0.622008467928146	 0.0446581987385205	 0.0446581987385205	  0.333333333333333	0.333333333333333	-0.333333333333333	-0.333333333333333	-0.0446581987385205	 -0.0446581987385205	-0.622008467928146	 -0.622008467928146	    -0.333333333333333	-0.333333333333333	-0.166666666666667	-0.166666666666667	 0.122008467928146	 0.122008467928146	-0.455341801261480	-0.455341801261480	-0.166666666666667	-0.166666666666667	-0.166666666666667	-0.166666666666667	  0.122008467928146	   0.122008467928146	-0.455341801261480	-0.455341801261480	-0.166666666666667	-0.166666666666667	0	0	                 0.288675134594813	 0.288675134594813	-0.288675134594813	-0.288675134594813	 0	                0;
                                         0	    0.333333333333333	-0.166666666666667	 0.166666666666667	-0.166666666666667	 0.166666666666667	-0.333333333333333	0	-0.288675134594813	0.0446581987385205	-0.455341801261480	   -0.122008467928146	-0.455341801261480	-0.122008467928146	-0.622008467928146	-0.288675134594813	 0.288675134594813	0.622008467928146	 0.122008467928146	 0.455341801261480   0.122008467928146	 0.455341801261480	-0.0446581987385205	 0.288675134594813	0	                0.333333333333333	-0.166666666666667	    0.166666666666667	-0.166666666666667	 0.166666666666667	 -0.333333333333333	0	                 0	                 0.333333333333333	-0.166666666666667	  0.166666666666667	    -0.166666666666667	  0.166666666666667	    -0.333333333333333	 0	                -0.288675134594813	 0.0446581987385205	-0.455341801261480	-0.122008467928146	-0.455341801261480	-0.122008467928146	-0.622008467928146	-0.288675134594813	 0.288675134594813	 0.622008467928146	  0.122008467928146	   0.455341801261480	 0.122008467928146	 0.455341801261480	-0.0446581987385205  0.288675134594813	0	0.333333333333333	-0.166666666666667	 0.166666666666667	-0.166666666666667	 0.166666666666667	-0.333333333333333	0;
                                         0	    0	                -0.288675134594813	-0.288675134594813	 0.288675134594813	 0.288675134594813	 0              	0	 0.166666666666667	0.166666666666667	-0.122008467928146     -0.122008467928146	 0.455341801261480	 0.455341801261480	 0.166666666666667	 0.166666666666667	 0.166666666666667	0.166666666666667	-0.122008467928146	-0.122008467928146	 0.455341801261480	 0.455341801261480	 0.166666666666667	 0.166666666666667	0.333333333333333	0.333333333333333	 0.0446581987385205 	0.0446581987385205	 0.622008467928146	 0.622008467928146	  0.333333333333333	0.333333333333333	-0.333333333333333	-0.333333333333333	-0.622008467928146	 -0.622008467928146	    -0.0446581987385205	 -0.0446581987385205	-0.333333333333333	-0.333333333333333	-0.166666666666667	-0.166666666666667	-0.455341801261480	-0.455341801261480	 0.122008467928146	 0.122008467928146	-0.166666666666667	-0.166666666666667	-0.166666666666667	-0.166666666666667	 -0.455341801261480	  -0.455341801261480	 0.122008467928146	 0.122008467928146	-0.166666666666667	-0.166666666666667	0	0	                -0.288675134594813	-0.288675134594813	 0.288675134594813	 0.288675134594813	 0	                0]);
        
        % Park-Transformation of the switchingstates factors
        Factors_d_q_x_y =single(zeros(4,1));
    
        Factors_d_q_x_y(3,1) = Factors_alpha_beta_x_y(3,Index);
        Factors_d_q_x_y(4,1) = Factors_alpha_beta_x_y(4,Index);
    
        cos_theta_el = single(cos(theta_el_with_offset));
        sin_theta_el = single(sin(theta_el_with_offset));
       
        Factors_d_q_x_y(1,1) = cos_theta_el*Factors_alpha_beta_x_y(1,Index)+sin_theta_el*Factors_alpha_beta_x_y(2,Index);
        Factors_d_q_x_y(2,1) = -sin_theta_el*Factors_alpha_beta_x_y(1,Index)+cos_theta_el*Factors_alpha_beta_x_y(2,Index);
    
        %Calculation of the voltages per switching state in alpha beta coordinates
        d_q_x_y_voltages_per_switching_state = single(u_dc_link_voltage*Factors_d_q_x_y);
    
        d_voltage_per_switching_state = d_q_x_y_voltages_per_switching_state(1,1);
        q_voltage_per_switching_state = d_q_x_y_voltages_per_switching_state(2,1);
        x_voltage_per_switching_state = d_q_x_y_voltages_per_switching_state(3,1);
        y_voltage_per_switching_state = d_q_x_y_voltages_per_switching_state(4,1);
    

end

== matlab function parallel_phase_voltages_per_switching_state_6/Phase_voltages_per_switching_state/Subsystem/MATLAB Function11 ==
  data: theta_el_with_offset input; d_voltage_per_switching_state output; u_dc_link_voltage input; Index input; q_voltage_per_switching_state output; x_voltage_per_switching_state output; y_voltage_per_switching_state output
function [d_voltage_per_switching_state, q_voltage_per_switching_state, x_voltage_per_switching_state, y_voltage_per_switching_state] = fcn(theta_el_with_offset, u_dc_link_voltage, Index)
      
        % Initial condition
            Index = Index+1+16;

    
        % Swichtingstates factors alpha beta x y
        Factors_alpha_beta_x_y = single([0	    0.333333333333333	-0.166666666666667	 0.166666666666667	-0.166666666666667	 0.166666666666667	-0.333333333333333	0	 0.288675134594813	0.622008467928146	 0.122008467928146  	0.455341801261480	 0.122008467928146	 0.455341801261480	-0.0446581987385205  0.288675134594813	-0.288675134594813	0.0446581987385205	-0.455341801261480	-0.122008467928146	-0.455341801261480	-0.122008467928146	-0.622008467928146	-0.288675134594813	0	                0.333333333333333	-0.166666666666667  	0.166666666666667	-0.166666666666667	 0.166666666666667	 -0.333333333333333	0	                 0	                 0.333333333333333	-0.166666666666667	  0.166666666666667	    -0.166666666666667	  0.166666666666667	    -0.333333333333333	 0	                 0.288675134594813	 0.622008467928146	 0.122008467928146	 0.455341801261480	 0.122008467928146	 0.455341801261480	-0.0446581987385205  0.288675134594813	-0.288675134594813	 0.0446581987385205  -0.455341801261480	  -0.122008467928146	-0.455341801261480	-0.122008467928146	-0.622008467928146	-0.288675134594813	0	0.333333333333333	-0.166666666666667	 0.166666666666667	-0.166666666666667	 0.166666666666667	-0.333333333333333	0;
                                         0	    0                    0.288675134594813	 0.288675134594813	-0.288675134594813	-0.288675134594813	 0	                0	 0.166666666666667	0.166666666666667	 0.455341801261480  	0.455341801261480	-0.122008467928146	-0.122008467928146	 0.166666666666667	 0.166666666666667	 0.166666666666667	0.166666666666667	 0.455341801261480   0.455341801261480	-0.122008467928146	-0.122008467928146	 0.166666666666667	 0.166666666666667	0.333333333333333	0.333333333333333	 0.622008467928146	    0.622008467928146	 0.0446581987385205	 0.0446581987385205	  0.333333333333333	0.333333333333333	-0.333333333333333	-0.333333333333333	-0.0446581987385205	 -0.0446581987385205	-0.622008467928146	 -0.622008467928146	    -0.333333333333333	-0.333333333333333	-0.166666666666667	-0.166666666666667	 0.122008467928146	 0.122008467928146	-0.455341801261480	-0.455341801261480	-0.166666666666667	-0.166666666666667	-0.166666666666667	-0.166666666666667	  0.122008467928146	   0.122008467928146	-0.455341801261480	-0.455341801261480	-0.166666666666667	-0.166666666666667	0	0	                 0.288675134594813	 0.288675134594813	-0.288675134594813	-0.288675134594813	 0	                0;
                                         0	    0.333333333333333	-0.166666666666667	 0.166666666666667	-0.166666666666667	 0.166666666666667	-0.333333333333333	0	-0.288675134594813	0.0446581987385205	-0.455341801261480	   -0.122008467928146	-0.455341801261480	-0.122008467928146	-0.622008467928146	-0.288675134594813	 0.288675134594813	0.622008467928146	 0.122008467928146	 0.455341801261480   0.122008467928146	 0.455341801261480	-0.0446581987385205	 0.288675134594813	0	                0.333333333333333	-0.166666666666667	    0.166666666666667	-0.166666666666667	 0.166666666666667	 -0.333333333333333	0	                 0	                 0.333333333333333	-0.166666666666667	  0.166666666666667	    -0.166666666666667	  0.166666666666667	    -0.333333333333333	 0	                -0.288675134594813	 0.0446581987385205	-0.455341801261480	-0.122008467928146	-0.455341801261480	-0.122008467928146	-0.622008467928146	-0.288675134594813	 0.288675134594813	 0.622008467928146	  0.122008467928146	   0.455341801261480	 0.122008467928146	 0.455341801261480	-0.0446581987385205  0.288675134594813	0	0.333333333333333	-0.166666666666667	 0.166666666666667	-0.166666666666667	 0.166666666666667	-0.333333333333333	0;
                                         0	    0	                -0.288675134594813	-0.288675134594813	 0.288675134594813	 0.288675134594813	 0              	0	 0.166666666666667	0.166666666666667	-0.122008467928146     -0.122008467928146	 0.455341801261480	 0.455341801261480	 0.166666666666667	 0.166666666666667	 0.166666666666667	0.166666666666667	-0.122008467928146	-0.122008467928146	 0.455341801261480	 0.455341801261480	 0.166666666666667	 0.166666666666667	0.333333333333333	0.333333333333333	 0.0446581987385205 	0.0446581987385205	 0.622008467928146	 0.622008467928146	  0.333333333333333	0.333333333333333	-0.333333333333333	-0.333333333333333	-0.622008467928146	 -0.622008467928146	    -0.0446581987385205	 -0.0446581987385205	-0.333333333333333	-0.333333333333333	-0.166666666666667	-0.166666666666667	-0.455341801261480	-0.455341801261480	 0.122008467928146	 0.122008467928146	-0.166666666666667	-0.166666666666667	-0.166666666666667	-0.166666666666667	 -0.455341801261480	  -0.455341801261480	 0.122008467928146	 0.122008467928146	-0.166666666666667	-0.166666666666667	0	0	                -0.288675134594813	-0.288675134594813	 0.288675134594813	 0.288675134594813	 0	                0]);
        
        % Park-Transformation of the switchingstates factors
        Factors_d_q_x_y =single(zeros(4,1));
    
        Factors_d_q_x_y(3,1) = Factors_alpha_beta_x_y(3,Index);
        Factors_d_q_x_y(4,1) = Factors_alpha_beta_x_y(4,Index);
    
        cos_theta_el = single(cos(theta_el_with_offset));
        sin_theta_el = single(sin(theta_el_with_offset));
       
        Factors_d_q_x_y(1,1) = cos_theta_el*Factors_alpha_beta_x_y(1,Index)+sin_theta_el*Factors_alpha_beta_x_y(2,Index);
        Factors_d_q_x_y(2,1) = -sin_theta_el*Factors_alpha_beta_x_y(1,Index)+cos_theta_el*Factors_alpha_beta_x_y(2,Index);
    
        %Calculation of the voltages per switching state in alpha beta coordinates
        d_q_x_y_voltages_per_switching_state = single(u_dc_link_voltage*Factors_d_q_x_y);
    
        d_voltage_per_switching_state = d_q_x_y_voltages_per_switching_state(1,1);
        q_voltage_per_switching_state = d_q_x_y_voltages_per_switching_state(2,1);
        x_voltage_per_switching_state = d_q_x_y_voltages_per_switching_state(3,1);
        y_voltage_per_switching_state = d_q_x_y_voltages_per_switching_state(4,1);
    

end
